simulink model "explicitaccel_microaccel"  (R2022b)
settings: Solver=FixedStepAuto  StartTime=0.0  StopTime=inf  FixedStep=0.05  RelTol=1e-3
undefined symbols (not defined in the file): Angular, Linear
libraries: robotlib x27
settings Model: Creator=ivory  LastModifiedBy=hayat
settings SolverCC: AlgebraicLoopSolver=TrustRegion
settings OptimizationCC: EnhancedBackFolding=on  PassReuseOutputArgsAs=Individual arguments  ZeroExternalMemoryAtStartup=off  ZeroInternalMemoryAtStartup=off  MaxStackSize=64  OptimizeBlockOrder=speed  DifferentSizesBufferReuse=on  OptimizationCustomize=off  EfficientTunableParamExpr=on
settings DebuggingCC: ParameterTunabilityLossMsg=error  UnconnectedInputMsg=warning  UnconnectedOutputMsg=warning  UnconnectedLineMsg=warning  SFMachineParentedDataDiag=warning
settings HardwareCC: ProdBitPerPointer=32  ProdBitPerSizeT=32  ProdBitPerPtrDiffT=32  ProdLargestAtomicFloat=None  ProdIntDivRoundTo=Undefined  ProdEndianess=Unspecified  ProdWordSize=32  ProdHWDeviceType=Generic->Unspecified (assume 32-bit Generic)
settings ModelReferenceCC: EnableRefExpFcnMdlSchedulingChecks=on
settings SFSimCC: MATLABDynamicMemAlloc=off  SimTargetLang=C++
settings RTWCC: Description=Embedded Coder  SystemTargetFile=ert.tlc  HardwareBoard=Robot Operating System (ROS)  TLCOptions="-aInlineSetEventsForThisBaseRateFcn=TLC_FALSE -aSuppressMultiTaskScheduler=TLC_FALSE  -aRateBasedStepFcn=0"  TemplateMakefile=ert_default_tmf  GenerateReport=on  Toolchain=Catkin  IncludeHyperlinkInReport=on  LaunchReport=on  TargetLang=C++  GenerateTraceInfo=on  GenerateTraceReport=on  GenerateTraceReportSl=on  GenerateTraceReportSf=on  GenerateTraceReportEml=on  DLArmComputeVersion=19.05
settings CodeAppCC: ForceParamTrailComments=on  IgnoreCustomStorageClasses=off  OperatorAnnotations=on  SimulinkDataObjDesc=on  SFDataObjDesc=on  InsertBlockDesc=on
settings ERTTargetCC: SupportContinuousTime=on  SupportVariableSizeSignals=on

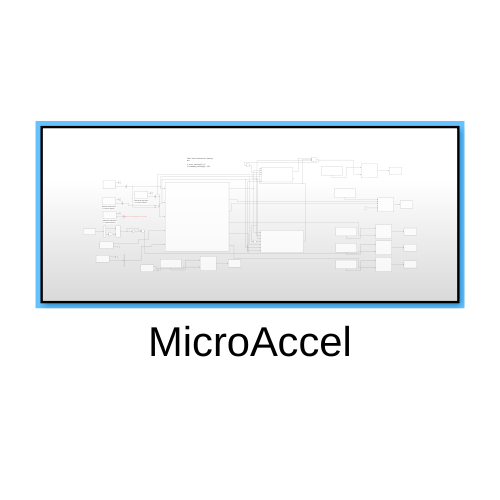
[thumbnail: Simulink's stored preview of the top-level diagram]
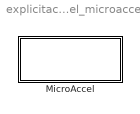
== system explicitaccel_microaccel ==
  MicroAccel : Subsystem

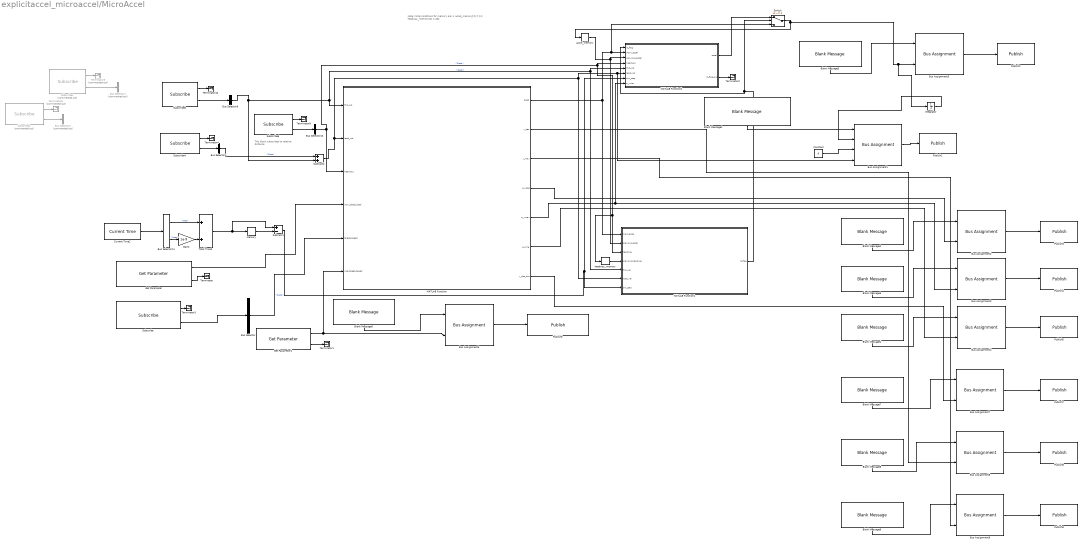
== system explicitaccel_microaccel/MicroAccel ==
  note: Note: initial conditions for memory are:
      |
      | 1. accel_memory[0] = 0
      | 2. headway_memory[0] = 252
  note: This block subscribes
      | to relative distance
  Blank Message1 : robotlib/Blank Message  messageClass=Message  entityType=geometry_msgs/Twist  messageType=geometry_msgs/Twist  SampleTime=inf  legacyBusStruct=off
  Blank Message{2..5,7..9} (7 alike) : robotlib/Blank Message  messageClass=Message  entityType=std_msgs/Float64  messageType=std_msgs/Float64  SampleTime=inf  legacyBusStruct=off
  Blank Message6 : robotlib/Blank Message  messageClass=Message  entityType=std_msgs/Bool  messageType=std_msgs/Bool  SampleTime=inf  legacyBusStruct=off
  Bus Assignment1 : BusAssignment  AssignedSignals=Linear.X,Angular.Z,Linear.Y
  Bus Assignment{2..9} (8 alike) : BusAssignment  AssignedSignals=Data
  Bus Selector{,4,9..10} (4 alike) : BusSelector  OutputSignals=Data
  Bus Selector1 : BusSelector  Commented=on  OutputSignals=Linear.X
  Bus Selector11 : BusSelector  OutputSignals=Sec,Nsec
  Bus Selector2 : BusSelector  Commented=on  OutputSignals=Linear.Z
  Constant : Constant  Value=0
  Current Time2 : robotlib/Current Time  OutputFormat=bus  SampleTime=-1  ModelName=explicitaccel_microaccel
  Gain2 : Gain  Gain=1e-9
  Get Parameter : robotlib/Get Parameter  ParameterSource=Specify your own  ParameterName=max_deaccel_lead  ParameterType=double  ParameterMaxArrayLength=16  ParameterInitialValue=-4.5  SampleTime=-1  ShowErrorCodeOutput=on  ModelName=explicitaccel_microaccel  BlockId=ParamGet_explicitaccel_microaccel_585
  Get Parameter1 : robotlib/Get Parameter  ParameterSource=Specify your own  ParameterName=use_target_speed  ParameterType=boolean  ParameterMaxArrayLength=16  ParameterInitialValue=0.0  SampleTime=-1  ShowErrorCodeOutput=on  ModelName=explicitaccel_microaccel  BlockId=ParamGet_explicitaccel_microaccel_631
  Integrator : Integrator
  MATLAB Function : MATLAB Function  TreatAsAtomicUnit=on
  MATLAB Function1 : MATLAB Function  TreatAsAtomicUnit=on
  MATLAB Function2 : MATLAB Function  TreatAsAtomicUnit=on
  Memory : Memory
  Publish1 : robotlib/Publish  topicSource=Specify your own  topic=cmd_vel  messageType=geometry_msgs/Twist  legacyBusStruct=off  messageQueueLength=1
  Publish2 : robotlib/Publish  topicSource=Specify your own  topic=cmd_accel  messageType=std_msgs/Float64  legacyBusStruct=off  messageQueueLength=1
  Publish3 : robotlib/Publish  topicSource=Specify your own  topic=a_vdesout  messageType=std_msgs/Float64  legacyBusStruct=off  messageQueueLength=1
  Publish4 : robotlib/Publish  topicSource=Specify your own  topic=a_vmaxout  messageType=std_msgs/Float64  legacyBusStruct=off  messageQueueLength=1
  Publish5 : robotlib/Publish  topicSource=Specify your own  topic=a_mngout  messageType=std_msgs/Float64  legacyBusStruct=off  messageQueueLength=1
  Publish6 : robotlib/Publish  topicSource=Specify your own  topic=targetspeedflag  messageType=std_msgs/Bool  legacyBusStruct=off  messageQueueLength=1
  Publish7 : robotlib/Publish  topicSource=Specify your own  topic=v_des_dot  messageType=std_msgs/Float64  legacyBusStruct=off  messageQueueLength=1
  Publish8 : robotlib/Publish  topicSource=Specify your own  topic=v_des  messageType=std_msgs/Float64  legacyBusStruct=off  messageQueueLength=1
  Publish9 : robotlib/Publish  topicSource=Specify your own  topic=v_max  messageType=std_msgs/Float64  legacyBusStruct=off  messageQueueLength=1
  Subscribe : robotlib/Subscribe  topicSource=Specify your own  topic=sp/target_speed  messageType=std_msgs/Float64  SampleTime=-1  legacyBusStruct=off  messageQueueLength=1
  Subscribe1 : robotlib/Subscribe  Commented=on  topicSource=Specify your own  topic=vel  messageType=geometry_msgs/Twist  SampleTime=-1  legacyBusStruct=off  messageQueueLength=1
  Subscribe2 : robotlib/Subscribe  Commented=on  topicSource=Specify your own  topic=rel_vel  messageType=geometry_msgs/Twist  SampleTime=-1  legacyBusStruct=off  messageQueueLength=1
  Subscribe4 : robotlib/Subscribe  topicSource=Specify your own  topic=rel_vel  messageType=std_msgs/Float64  SampleTime=-1  legacyBusStruct=off  messageQueueLength=1
  Subscribe6 : robotlib/Subscribe  topicSource=Specify your own  topic=lead_dist  messageType=std_msgs/Float64  SampleTime=-1  legacyBusStruct=off  messageQueueLength=1
  Subscribe8 : robotlib/Subscribe  topicSource=Specify your own  topic=vel  messageType=std_msgs/Float64  SampleTime=-1  legacyBusStruct=off  messageQueueLength=1
  Subtract1 : Sum  Inputs=+-
  Subtract2 : Sum
  Switch : Switch  Criteria=u2 ~= 0  SaturateOnIntegerOverflow=off  InputSameDT=off
  Terminator{,1..4,9..10} (7 alike) : Terminator
  Terminator5 : Terminator  Commented=on
  Terminator6 : Terminator  Commented=on
  Total Time2 : Sum
  accel_memory : Memory
  headway_memory : Memory  InitialCondition=252
  wires:
  Subscribe8/1 -> Terminator10/1
  Subscribe8/2 -> Bus Selector9/1
  Bus Selector9/1 -> MATLAB Function1/5(this_vel), MATLAB Function2/5(this_vel), MATLAB Function/1(this_vel), Subtract2/2  "<Data>"
  Subscribe6/1 -> Terminator9/1
  Subscribe6/2 -> Bus Selector10/1
  Bus Selector10/1 -> headway_memory/1, MATLAB Function1/3(headway), MATLAB Function2/4(headway), MATLAB Function/3(headway)  "<Data>"
  Bus Selector11/1 -> Total Time2/1  "<Sec>"
  Gain2/1 -> Total Time2/2
  Bus Selector11/2 -> Gain2/1  "<Nsec>"
  Total Time2/1 -> Subtract1/1, Memory/1
  Current Time2/1 -> Bus Selector11/1
  Memory/1 -> Subtract1/2
  Subtract1/1 -> MATLAB Function2/7(sim_step), MATLAB Function1/7(sim_step)
  Get Parameter/2 -> Terminator/1
  Get Parameter/1 -> MATLAB Function/4(max_decel_lead)
  Constant/1 -> Bus Assignment1/3
  Bus Assignment1/1 -> Publish1/1
  Blank Message1/1 -> Bus Assignment1/1
  MATLAB Function/3(v_max) -> Bus Assignment9/2
  MATLAB Function/5(a_vmax) -> Bus Assignment3/2, MATLAB Function2/8(a_vmax)
  MATLAB Function/2(v_des) -> Bus Assignment8/2
  Subscribe/1 -> Terminator3/1
  Subscribe/2 -> Bus Selector/1
  Bus Selector/1 -> MATLAB Function/5(target_speed)  "<Data>"
  Blank Message2/1 -> Bus Assignment2/1
  MATLAB Function/4(a_vdes) -> Bus Assignment2/2
  Blank Message3/1 -> Bus Assignment3/1
  Blank Message4/1 -> Bus Assignment4/1
  Blank Message5/1 -> Bus Assignment5/1
  MATLAB Function/1(accel) -> MATLAB Function1/1(main_accel), Switch/3, MATLAB Function2/2(main_accel)
  Bus Assignment5/1 -> Publish2/1
  Bus Assignment2/1 -> Publish3/1
  Bus Assignment3/1 -> Publish4/1
  Bus Assignment4/1 -> Publish5/1
  MATLAB Function/6(a_mng) -> Bus Assignment4/2
  Bus Selector4/1 -> Subtract2/1  "<Data>"
  Subscribe4/2 -> Bus Selector4/1
  Subscribe4/1 -> Terminator4/1
  Subtract2/1 -> MATLAB Function1/6(lead_vel), Bus Assignment1/4, MATLAB Function2/6(lead_vel), MATLAB Function/2(lead_vel)
  Get Parameter1/2 -> Terminator1/1
  Bus Assignment6/1 -> Publish6/1
  Get Parameter1/1 -> MATLAB Function/6(use_target_speed), Bus Assignment6/2
  Blank Message6/1 -> Bus Assignment6/1
  MATLAB Function1/1(lc_flag) -> Switch/2, MATLAB Function2/1(lc_flag)
  accel_memory/1 -> MATLAB Function1/2(previous_accel), MATLAB Function2/3(previous_accel)
  headway_memory/1 -> MATLAB Function1/4(previous_headway)
  MATLAB Function2/1(accel) -> Switch/1
  Switch/1 -> Integrator/1, Bus Assignment5/2, accel_memory/1
  MATLAB Function2/2(lc_flag_out) -> Terminator2/1
  Bus Assignment7/1 -> Publish7/1
  Blank Message7/1 -> Bus Assignment7/1
  MATLAB Function/7(v_des_dot) -> Bus Assignment7/2
  Blank Message8/1 -> Bus Assignment8/1
  Bus Assignment8/1 -> Publish8/1
  Bus Assignment9/1 -> Publish9/1
  Blank Message9/1 -> Bus Assignment9/1
  Subscribe1/2 -> Bus Selector1/1
  Subscribe1/1 -> Terminator5/1
  Subscribe2/1 -> Terminator6/1
  Subscribe2/2 -> Bus Selector2/1
  Integrator/1 -> Bus Assignment1/2

== matlab function explicitaccel_microaccel/MicroAccel/MATLAB Function1 ==
  data: main_accel input; lc_flag output; previous_accel input; headway input; previous_headway input; this_vel input; lead_vel input; sim_step input
function lc_flag = detect_lane_change(main_accel, previous_accel, headway, previous_headway, this_vel, lead_vel, sim_step)
    lc_thresh = 3.5;
    a_comfort = 0.9 * sim_step;
    th_safe = 2;
    ttc_safe = 4.5;

    rv = lead_vel - this_vel;
    da = abs(main_accel - previous_accel);
    
    th = (this_vel > 0) * (headway / this_vel) + (this_vel <= 0) * 60;
    ttc = (rv < 0) * (-headway / rv) +  (rv >= 0) *  60;
    difference = headway - previous_headway;

    if difference <= -lc_thresh
        if da > a_comfort
            if rv >= 0 && th > th_safe
                lc_flag = -1;
                return
            elseif rv < 0 && ttc > ttc_safe
                lc_flag = -1;
                return
            end 
        end 
    elseif difference >= lc_thresh
        if da > a_comfort
            if rv >= 0 && th > th_safe
                lc_flag = 1; 
                return
            elseif rv < 0 && ttc > ttc_safe
                lc_flag = 1; 
                return
            end 
        end
    end 

    lc_flag = 0; 
end

== matlab function explicitaccel_microaccel/MicroAccel/MATLAB Function ==
  settings: updateMethod=DISCRETE
  data: this_vel input; lead_vel input; accel output; v_des output; v_max output; headway input; max_decel_lead input; target_speed input; a_vdes output; a_vmax output; a_mng output; use_target_speed input; v_des_dot output
function [accel, v_des,v_max, a_vdes,a_vmax,a_mng, v_des_dot] =  get_main_accel_2(this_vel, lead_vel, headway, max_decel_lead, target_speed, use_target_speed)
        

    %% model parameters
    max_accel = 1; %Max acceleration
    max_decel_des = -0.4;
    max_decel = -3; %Max decceleration (safety wise)
    max_decel_comfort = -1; %Max confortable decceleration (i.e. not for safety)
    gap_pen = 1;
    in_head = 2;
    gap_target = 2;
    v_limit = 30;
    v_hist = 20;
    period = 128; 
    long_time_head = 5;
    target_time_head = 3;
    h0=2.5;
    s0=18;
    k = 1; 
    sim_step = 0.05;
    average_step = floor(period./sim_step);
    length_acc_avg = floor(1./sim_step);
    h1= target_time_head.*this_vel;
    
    if(~use_target_speed) | target_speed == 0
        target_speed = -1;
    end

    %treat lead_vel to keep 0 as no signal
    if lead_vel == 0
        lead_vel = 0.2;
    end


        % Declare persistent variables
        persistent previous_v_des;
        persistent previous_v_max;
        persistent previous_dx;
        persistent previous_lead_acc;
        persistent prev_vels
        persistent t_length 
        persistent no_initial_signal
        persistent prev_lead_acc
        persistent t_length_acc
        persistent previous_lead_vel_real

        
        if isempty(previous_v_des)
            t_length = 1;
            previous_v_des = NaN;
            previous_v_max = NaN;
            previous_dx = NaN;
            previous_lead_acc = NaN;
            previous_lead_vel_real = NaN;
            prev_vels = zeros(1, average_step);
            prev_vels(average_step)= lead_vel;
            no_initial_signal = 0;
        else
            prev_vels = [prev_vels(2:end),lead_vel];
            t_length = nnz(prev_vels);
        end
        
        % in order to deal with ZeroDivisionError
        if abs(headway) < 1e-3
            headway = 1e-3;
        end

        %Avoiding loss of signal
        if headway >= 252 && isnan(previous_dx)
           %previous_dx remains NaN until no_initial_signal = 0 again.
           no_initial_signal = 1;
           % No recording before getting a signal
           prev_vels(average_step) = 0;
           t_length = nnz(prev_vels);
           assert(t_length == 0) 
        elseif headway <252
            no_initial_signal =0;
        elseif headway >= 252
           %Don't store with velocity but still flush the memory and keep a
           %0 to indicate the loss of signal
           prev_vels(end) = 0;
           assert(length(prev_vels)==average_step)
           t_length = nnz(prev_vels);
           lead_vel = previous_lead_vel_real; 
            if previous_dx < 220
                %computing new effective velocity
                headway = previous_dx +in_head.*sim_step;          
            end
        end

        %Update previous lead vel
        previous_lead_vel_real = lead_vel;


        % TODO (Amaury & Shengquan): update as needed
        if target_speed == -1
            ref_vel = 35;
            if t_length == 0
                target_speed = v_limit;
            else
                target_speed = sum(prev_vels)/t_length;
            end
            assert(target_speed>=0)

            target_speed = min((0.1.*max(0,1.*(headway-max(h1,30))./max(1, this_vel))^2+ target_speed),ref_vel); %%%%%%%%%Penalise too large headway, the constants can be modified
        else
            ref_vel = 35;
            target_speed = max(min(target_speed, 1.2.*lead_vel), 0.8*min(lead_vel,ref_vel));
            if no_initial_signal == 0                 
                target_speed = max(min(target_speed, 1.2.*lead_vel), 0.8*min(lead_vel,ref_vel));
            end
        end

        % Create leader's accel
        if prev_vels(end-1) == 0 | prev_vels(end) == 0 | no_initial_signal == 1 %Warning what when the vehicle is really stopped, this should not happen
            lead_acc = 0;
        elseif (lead_vel - prev_vels(end-1)) < 3.3 * sim_step
            lead_acc = (lead_vel - prev_vels(end-1)) / sim_step;
        else
            lead_acc = previous_lead_acc;
        end

        previous_lead_acc = lead_acc;  % Update lead_acc for next timestep

        % Create the acceleration
        % TODO add the patch for spotting the lack of signal.
        % TODO maybe issues when there is a lead veh then no lead veh then again a lead veh for the memory quantity

        % Create v_des from the motion planner

        v_des = target_speed;
        assert(v_des ~= -1);
        if isnan(previous_v_des)  % Initial step
            v_des_dot = 0;
        else
            %v_des_dot = (v_des - previous_v_des ) / sim_step;  % Create the derivative of V_DES
            v_des_dot = 0;
        end
        
        % update previous v_des
        previous_v_des = v_des;



        if isnan(lead_vel) | (headway == 252 && previous_dx> 220) | no_initial_signal == 1    % no car ahead % TODO: Put this before in case no veh in front Adapt in matlab?
            a_mng = max_accel;
            v_max_dot = 0;
            v_max = v_limit;
            if isnan(lead_vel) | no_initial_signal == 1
                v_des = v_limit;
                v_des_dot = 0;
                previous_v_des = v_limit;
            end
        else
            dx = headway;
            if isnan(previous_dx)  % Initial step
                previous_dx = dx;
            end
            % Compute v_max and its derivative
            v_max = sqrt(2 * abs(max_decel) * (max(dx - s0, 0) + 0.5 * ((lead_vel)^ 2) / abs(max_decel_lead)));

            if isnan(previous_v_max)  % Initial step
                v_max_dot = 0;
            elseif abs(dx - previous_dx) > sim_step * 50  % Exclude the discontinuities in headway
                v_max_dot = 0;
            else
                v_max_dot = (v_max - previous_v_max) / sim_step;  % Compute the derivative of v_max
            end
            previous_v_max = v_max;  % update previous_v_max



            %Create an average of the lead acc
            if isempty(prev_lead_acc) %Initial step
               prev_lead_acc = zeros(1,length_acc_avg);
               prev_lead_acc(length_acc_avg) = lead_acc;
            else
                prev_lead_acc = [prev_lead_acc(2:end),lead_acc];
            end
            t_length_acc = nnz(prev_lead_acc);
            if t_length_acc == 0
                lead_acc_avg = 0;
            else
                lead_acc_avg = sum(prev_lead_acc)/t_length_acc;
            end

            % Compute a_mng (acceleration managment)

            if lead_acc_avg < 0
                a_0 = lead_acc_avg * this_vel / (lead_vel + 0.001);
                a_12 = -0.5* (this_vel).^ 2/ (max(0, dx - s0) + 0.5 * ((lead_vel + 0.00001).^ 2)/abs(lead_acc_avg - 0.01));
                if a_0 < a_12
                    a_mng = a_12;
                else
                    if lead_vel >= this_vel
                        a_mng = a_0;
                    else
                        a_mng = lead_acc_avg - ((lead_vel - this_vel) ^ 2) / ( 2 * max(dx -s0, 0.001) );
                    assert(a_mng <= 0);  % changed to <= 0
                    end
                end
            elseif lead_acc_avg >= 0
                if lead_vel <= this_vel
                    a_mng = lead_acc_avg - ((max(0, this_vel - lead_vel)) ^ 2) / ( 2 * max(dx - s0, 0.001) );
                else
                    a_mng = min(max_accel, lead_acc_avg + (lead_acc_avg) * (lead_vel - this_vel));
                    % TODO this can be changed / might be the source of some oscillations. together with long time head
                end
            else
                a_mng = NaN;
                fprintf("This is an error\n");
            end

            % Deactivate a_mng when the vehicle is above a certain distance
            assert(long_time_head > 1);
            assert(long_time_head > gap_target);


            if dx > this_vel * (long_time_head - 1)
                a_mng = a_mng + gap_pen * (dx - (long_time_head - 1) * this_vel) / max(this_vel, 0.01);
            end

           previous_dx = dx;  % Update the previous headway 
        end
        a_mng = max(a_mng, -abs(max_decel_comfort));


        % Final acceleration
        a_vdes = max( -k * (this_vel - v_des) + v_des_dot, -abs(max_decel_des));
        a_vmax = -k * (this_vel - v_max) + v_max_dot;
        accel = min(min(a_vdes, a_vmax), a_mng);
        accel = min(max(accel, -abs(max_decel)), max_accel);

        if this_vel >= v_limit
            accel = min(0, accel);
        end
end

== matlab function explicitaccel_microaccel/MicroAccel/MATLAB Function2 ==
  data: lc_flag input; accel output; main_accel input; previous_accel input; headway input; this_vel input; lead_vel input; sim_step input; lc_flag_out output; a_vmax input
function [accel, lc_flag_out] = get_lc_recovery_accel(lc_flag, ...
                               main_accel, previous_accel, ...
                               headway, this_vel, lead_vel, sim_step,...
                               a_vmax)
    h_star = 1.32;
    rv_star_positive = 1;
    rv_star_negative = 10.34/headway; 
    epsilon = 0.3 * sim_step;
    f_h = 0.75;
    f_rv = 0.25;
    
    th = (this_vel > 0) * (headway / this_vel) + (this_vel <= 0) * 60;
    rv = lead_vel - this_vel; 
    rv_star = rv_star_positive * (rv >= 0) + rv_star_negative * (rv < 0);
    
    alpha = f_h * tanh(h_star * th) + f_rv * (0.5 * tanh(rv_star * rv) + 0.5);
    recovery_accel = alpha * previous_accel + (1 - alpha) * main_accel;
    
    if abs(recovery_accel - main_accel) < epsilon
        accel = main_accel; 
        lc_flag_out = 0; 
    else
        accel = recovery_accel; 
        lc_flag_out = lc_flag; 
    end
    accel = min(accel,a_vmax);
end
